simulink model "Modelo_Balancin"  (R2021a)
settings: Solver=VariableStepAuto  StartTime=0.0  StopTime=20.0  RelTol=1e-3
model workspace (MAT data in the model file):
  deno = [1 1.774 3.15]
values from neighbouring files (symbols this model uses):
  gr = 57.2958    [Funciones.m]
  h = 8.42e-3    (= 0.00842)    [Funciones.m]
  V_T = 0.02    [Funciones.m]
undefined symbols (not defined in the file or in its folder): Denominator, Numerador
settings Model: Creator=facun  LastModifiedBy=facun

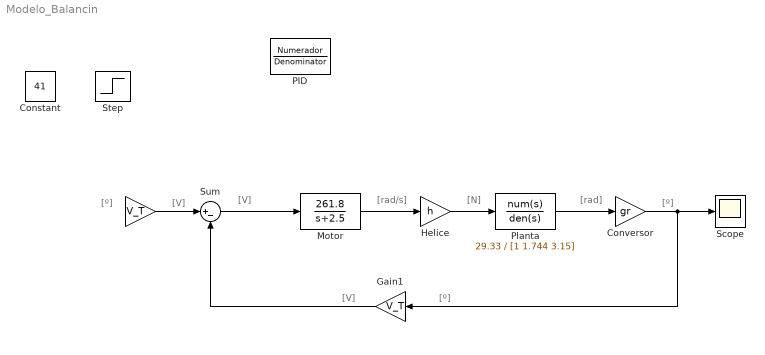
== system Modelo_Balancin ==
  note: [º]
  note: [rad/s]
  note: [V]
  note: [V]
  note: [N]
  note: [rad]
  note: [º]
  note: [º]
  note: [V]
  " " : Gain  Gain=V_T
  Constant : Constant  Value=41
  Conversor : Gain  Gain=gr
  Gain1 : Gain  Gain=V_T
  Helice : Gain  Gain=h
  Motor : TransferFcn  Numerator=261.8  Denominator=[1 2.5]
  PID : TransferFcn  Numerator=Numerador  Denominator=Denominator
  Planta : TransferFcn  Numerator=29.33  Denominator=[1 1.744 3.15]
  Scope : Scope
  Step : Step  Time=20  SampleTime=0
  Sum : Sum  Inputs=|+-
  wires:
  Motor/1 -> Helice/1
  Helice/1 -> Planta/1
  Planta/1 -> Conversor/1
  Conversor/1 -> Gain1/1, Scope/1
  " "/1 -> Sum/1
  Sum/1 -> Motor/1
  Gain1/1 -> Sum/2
